simulink model "DC_motor_position"  (R2018a)
settings: Solver=ode15s  StartTime=0.0  StopTime=0.5  RelTol=1e-3
values from neighbouring files (symbols this model uses):
  b = 3.5077E-6    (= 3.5077e-06)    [DC_motor_position.m]    (also in DC_motor_speed_para.m = 0.1; cruise_control_para.m = 50)
  J = 3.2284E-6    (= 3.2284e-06)    [DC_motor_position.m]    (also in DC_motor_speed_para.m = 0.01)
  K = 0.0274    [DC_motor_position.m]
  L = 2.75E-6    (= 2.75e-06)    [DC_motor_position.m]    (also in DC_motor_speed_para.m = 0.5)
  R = 4    [DC_motor_position.m]    (also in DC_motor_speed_para.m = 1)
settings Model: Creator=Infi  LastModifiedBy=Infi

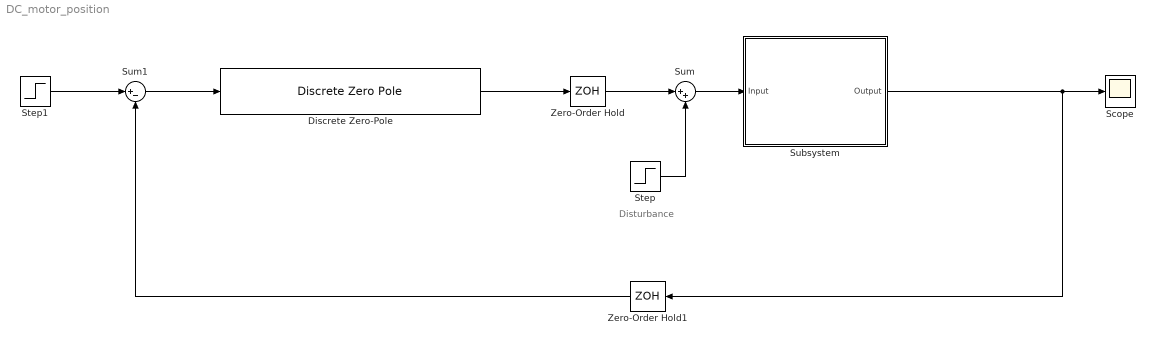
== system DC_motor_position ==
  note: Disturbance
  Discrete Zero-Pole : DiscreteZeroPole  Zeros=[0.95 0.8 0.8]  Poles=[-0.98 0.6 1]  Gain=100  SampleTime=0.001
  Scope : Scope
  Step : Step  Time=0.03  SampleTime=0
  Step1 : Step  Time=0  SampleTime=0.001
  Subsystem : Subsystem
  Sum : Sum  Inputs=|++
  Sum1 : Sum  Inputs=|+-
  Zero-Order Hold : ZeroOrderHold  SampleTime=0.001
  Zero-Order Hold1 : ZeroOrderHold  SampleTime=0.001
  wires:
  Discrete Zero-Pole/1 -> Zero-Order Hold/1
  Step/1 -> Sum/2
  Zero-Order Hold/1 -> Sum/1
  Sum/1 -> Subsystem/1(Input)
  Sum1/1 -> Discrete Zero-Pole/1
  Step1/1 -> Sum1/1
  Subsystem/1(Output) -> Scope/1, Zero-Order Hold1/1
  Zero-Order Hold1/1 -> Sum1/2

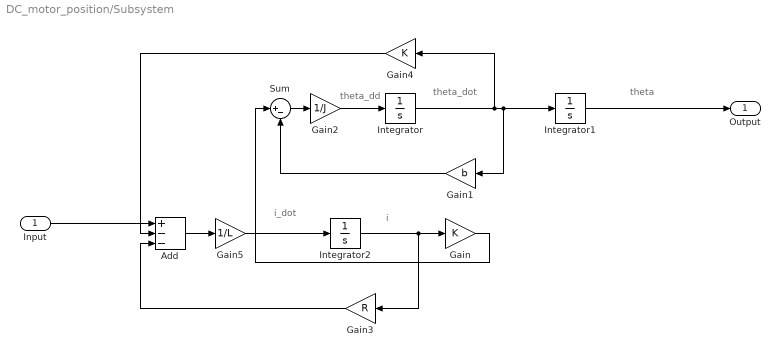
== system DC_motor_position/Subsystem ==
  note: i_dot
  note: i
  note: theta
  note: theta_dd
  note: theta_dot
  Input : Inport
  Add : Sum  Inputs=+--
  Gain : Gain  Gain=K
  Gain1 : Gain  Gain=b
  Gain2 : Gain  Gain=1/J
  Gain3 : Gain  Gain=R
  Gain4 : Gain  Gain=K
  Gain5 : Gain  Gain=1/L
  Integrator : Integrator
  Integrator1 : Integrator
  Integrator2 : Integrator
  Sum : Sum  Inputs=|+-
  Output : Outport
  wires:
  Gain2/1 -> Integrator/1
  Sum/1 -> Gain2/1
  Gain3/1 -> Add/3
  Gain/1 -> Sum/1
  Integrator/1 -> Gain4/1, Gain1/1, Integrator1/1
  Gain1/1 -> Sum/2
  Integrator1/1 -> Output/1
  Input/1 -> Add/1
  Integrator2/1 -> Gain3/1, Gain/1
  Gain4/1 -> Add/2
  Add/1 -> Gain5/1
  Gain5/1 -> Integrator2/1
